simulink model "Lab7Transmitancja"  (R2018a)
settings: Solver=VariableStepAuto  StartTime=0.0  StopTime=50.0  MaxStep=0.001  RelTol=1e-3
undefined symbols (not defined in the file or in its folder): delay, h10, h20, U, Yf11, Yf12, Yf21, Yf22
settings Model: Creator=aplov  LastModifiedBy=aplov

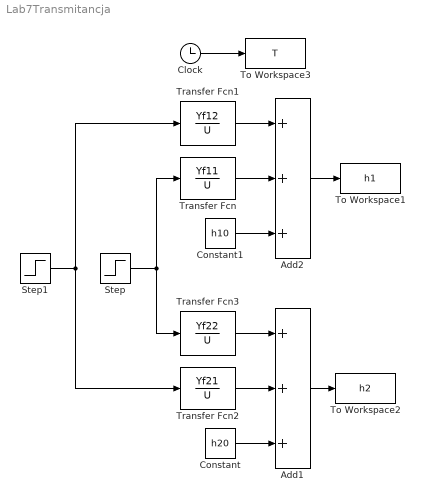
== system Lab7Transmitancja ==
  Add1 : Sum  Inputs=+++
  Add2 : Sum  Inputs=+++
  Clock : Clock
  Constant : Constant  Value=h20
  Constant1 : Constant  Value=h10
  Step : Step  Time=delay  SampleTime=0
  Step1 : Step  Time=delay  SampleTime=0
  To Workspace1 : ToWorkspace  VariableName=h1  SampleTime=-1
  To Workspace2 : ToWorkspace  VariableName=h2  SampleTime=-1
  To Workspace3 : ToWorkspace  VariableName=T  SampleTime=-1
  Transfer Fcn : TransferFcn  Numerator=Yf11  Denominator=U
  Transfer Fcn1 : TransferFcn  Numerator=Yf12  Denominator=U
  Transfer Fcn2 : TransferFcn  Numerator=Yf21  Denominator=U
  Transfer Fcn3 : TransferFcn  Numerator=Yf22  Denominator=U
  wires:
  Add1/1 -> To Workspace2/1
  Transfer Fcn2/1 -> Add1/2
  Transfer Fcn3/1 -> Add1/1
  Clock/1 -> To Workspace3/1
  Constant/1 -> Add1/3
  Transfer Fcn1/1 -> Add2/1
  Transfer Fcn/1 -> Add2/2
  Constant1/1 -> Add2/3
  Add2/1 -> To Workspace1/1
  Step/1 -> Transfer Fcn/1, Transfer Fcn3/1
  Step1/1 -> Transfer Fcn2/1, Transfer Fcn1/1
